simulink model "HarmMultisine_sim"  (R2019b)
settings: Solver=VariableStepAuto  StartTime=0.0  StopTime=10.0  RelTol=1e-3
settings Model: Creator=s164234  LastModifiedBy=s164234

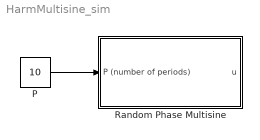
== system HarmMultisine_sim ==
  P : Constant  Value=10
  "Random Phase Multisine " : Subsystem
  wires:
  P/1 -> "Random Phase Multisine "/1("P (number of periods) ")

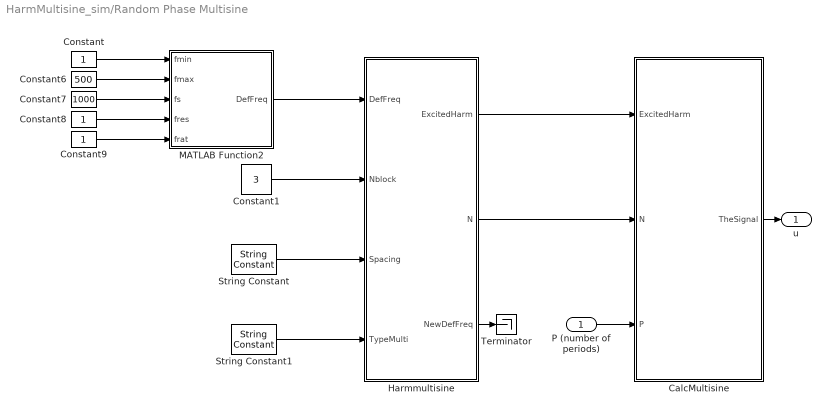
== system HarmMultisine_sim/Random Phase Multisine  ==
  "P (number of periods) " : Inport
  "CalcMultisine " : MATLAB Function  TreatAsAtomicUnit=on
  Constant : Constant
  Constant1 : Constant  Value=3
  Constant6 : Constant  Value=500
  Constant7 : Constant  Value=1000
  Constant8 : Constant
  Constant9 : Constant
  "Harmmultisine " : MATLAB Function  TreatAsAtomicUnit=on
  MATLAB Function2 : MATLAB Function  TreatAsAtomicUnit=on
  String Constant : StringConstant  String='log'
  String Constant1 : StringConstant  String='full'
  Terminator : Terminator
  u : Outport
  wires:
  "Harmmultisine "/2(N) -> "CalcMultisine "/2(N)
  Constant9/1 -> MATLAB Function2/5(frat)
  String Constant1/1 -> "Harmmultisine "/4(TypeMulti)
  Constant1/1 -> "Harmmultisine "/2(Nblock)
  Constant/1 -> MATLAB Function2/1(fmin)
  Constant7/1 -> MATLAB Function2/3(fs)
  String Constant/1 -> "Harmmultisine "/3(Spacing)
  "CalcMultisine "/1(TheSignal) -> u/1
  Constant6/1 -> MATLAB Function2/2(fmax)
  "Harmmultisine "/1(ExcitedHarm) -> "CalcMultisine "/1(ExcitedHarm)
  Constant8/1 -> MATLAB Function2/4(fres)
  MATLAB Function2/1(DefFreq) -> "Harmmultisine "/1(DefFreq)
  "P (number of periods) "/1 -> "CalcMultisine "/3(P)
  "Harmmultisine "/3(NewDefFreq) -> Terminator/1

== matlab function HarmMultisine_sim/Random Phase Multisine /Harmmultisine  ==
  data: DefFreq input; ExcitedHarm output; Nblock input; Spacing input; TypeMulti input; N output; NewDefFreq output
function [ExcitedHarm, N, NewDefFreq] = HarmMultisine(DefFreq, Nblock, Spacing, TypeMulti)
%
%       function [ExcitedHarm, N, NewDefFreq] = HarmMultisine(DefFreq, Nblock, Spacing, TypeMulti);
%
%       calculates the harmonic content of an odd or full random harmonic grid multisine signal
%       with a linear or a logarithmic spacing in the band defined by [fmin, fmax]
%       for a lowpass design
%           fmin = fres/2	for odd multisines
%           fmin = fres     for full multisines
%       where
%           fres =          the frequency spacing between two consecutive odd harmonics for odd multisines 
%           fres =          the frequency spacing between two consecutive harmonics for full multisines 
%
%
%   OUTPUT
%
%       ExcitedHarm     =   excited frequencies of the multisine expressed in harmonic numbers
%
%       N               =   number of time domain samples in one period
%
%       NewDefFreq      =   struct containing the information about the sampling frequency, frequency resolution,
%                           and the excited frequency band {'fs', 'fmin', 'fmax', 'fres', 'frat'}
%                               NewDefFreq.fs      =    sampling frequency of the generator (remains unchanged!)
%                               NewDefFreq.fres    =    frequency spacing in Hz between the (odd) harmonics 
%                                                       fres is modified such that fs/fres is an integer number
%                                                       Note: not all (odd) harmonics are excited; especially for the log spacing
%                               NewDefFreq.fmin    =    lowest excited frequency in Hz
%                                                       fmin is modified such that fmin/fres is an (odd) integer number
%                                                       (for lowpass design fmin = fres/2)
%                               NewDefFreq.fmax    =    largest excited frequency in Hz
%                                                       fmax is modified such that fmax/fres is an (odd) integer number
%
%   INPUT
%
%       DefFreq         =   struct containing the information about the sampling frequency, frequency resolution,
%                           and the excited frequency band {'fs', 'fmin', 'fmax', 'fres', 'frat'}
%                               DefFreq.fs      =   sampling frequency of the generator
%                               DefFreq.fres    =   frequency spacing in Hz between the (odd) harmonics 
%                               DefFreq.fmin    =   lowest excited frequency in Hz
%                                                   (for lowpass design of odd multisines fmin = fres/2)
%                               DefFreq.fmax    =   largest excited frequency in Hz
%                               DefFreq.frat    =   ratio between consecutive (odd) harmonics for a logarithmic frequency spacing
%
%       Nblock          =   size of the group of consecutive (odd) harmonics where one is randomly eliminated
%                           if Nblock = Inf then no detection lines are present 
%
%       Spacing         =   linear or logarithmic frequency spacing; optional parameter (default = 'linear') 
%                               'lin', 'linear':       linear frequency spacing
%                               'log', 'logarithmic':  quasi logarithmic frequency spacing (rounded to DFT grid)
%
%       TypeMulti       =   type multisine; optional (default = 'odd')
%                               'odd':   odd random harmonic grid multisine        
%                               'full':  full random harmonic grid multisine 
%
% Copyright (c) Rik Pintelon, Vrije Universiteit Brussel - dept. ELEC, March 2006 
% All rights reserved.
% Software can be used freely for non-commercial applications only.
% Version 4 December 2007
%

%%%%%%%%%%%%%%%%%%%%%%%%%%%%
% initialize the variables %
%%%%%%%%%%%%%%%%%%%%%%%%%%%%

fs = DefFreq.fs;
fres = DefFreq.fres;
fmin = DefFreq.fmin;
fmax = DefFreq.fmax;

if isfield(DefFreq, 'frat')
	if ~isempty(DefFreq.frat)
        frat = DefFreq.frat;
	end % if not empty
end % if isfield

% type of the frequency spacing
if nargin == 2
    Spacing = 'lin';
end % if
Spacing = lower(Spacing);

% type of the multisine
if nargin <= 3
    TypeMulti = 'odd';
end % if
TypeMulti = lower(TypeMulti);


%%%%%%%%%%%%%%%%%%%%%%%%%%%%%%%%%%%%%%%%
% calculation odd random harmonic grid %
%%%%%%%%%%%%%%%%%%%%%%%%%%%%%%%%%%%%%%%%

if strcmp(TypeMulti, 'odd')
    fres = fres/2;                  % frequency spacing between odd and even harmonics
end % if odd multisine
N = ceil(fs/fres);                  % number of time domain points in one period
fres = fs/N;
FreqSpan = floor(fmax/fres);        % frequency span for a lowpass signal

% calculate the (odd) random harmonic numbers for a lowpass signal
switch Spacing
    
    case {'lin', 'linear'}				
		ExcitedHarm = lintone(FreqSpan, Nblock, TypeMulti);
		
    case {'log', 'logarithmic'}
        ExcitedHarm = logtone(FreqSpan, frat, Nblock, TypeMulti);
        
end % switch Spacing

% convert lowpass in bandpass
FirstNonZeroHarm = ceil(fmin/fres);
RemoveHarm = find(ExcitedHarm < FirstNonZeroHarm);
ExcitedHarm(RemoveHarm) = [];


%%%%%%%%%%%%%%%%%%%%%%%%
% realised frequencies %
%%%%%%%%%%%%%%%%%%%%%%%%

NewDefFreq.fs = fs;
NewDefFreq.fres = fres;
if strcmp(TypeMulti, 'odd')
    NewDefFreq.fres = 2*NewDefFreq.fres;       % frequency spacing between the odd harmonics
end % if odd multisine
NewDefFreq.fmin = ExcitedHarm(1)*fres;
NewDefFreq.fmax = ExcitedHarm(end)*fres;

function ExcitedHarm = logtone(FreqSpan, FreqRatio, Nblock, TypeMulti);
%
%	ExcitedHarm = logtone(FreqSpan, FreqRatio, Nblock, TypeMulti);
%
%		(odd) multisine with logaritmic frequency distribution and randomly
%		distributed (odd) detection lines.
%		calculates a logarithmic distributed frequency grid of (odd) harmonics
%		where one (odd) harmonic out of Nblock consecutive harmonics is left out		
%
%	OUTPUT PARAMETERS
%
%		ExcitedHarm		= vector containing the excited harmonics
%
%	INPUT PARAMETERS
%
%		FreqSpan		=   ratio fmax/fmin
%		FreqRatio		=   ratio consecutive odd frequencies in logtone
% 		Nblock			=   number of lines per block
%                           if Nblock = Inf then no detection lines are present 
%       TypeMulti       =   type multisine; optional (default = 'odd')
%                               'odd':   odd random harmonic grid multisine        
%                               'full':  full random harmonic grid multisine 
%
% Johan Schoukens and Rik Pintelon, September 2003
% Version March 18, 2008
%

% type of the multisine
if nargin == 3
    TypeMulti = 'odd';
end % if
TypeMulti = lower(TypeMulti);

% selection of the frequency span
switch TypeMulti    
    case 'odd', Fmax = FreqSpan/2;
    case 'full', Fmax = FreqSpan;        
end % switch

% resolution of the frequency axis = fmin 
% => total number of frequencies on the linear grid = FreqSpan = fmax/fmin

freqv = [1:Fmax];
ExcitedHarm = lin2log(freqv, FreqRatio);		% generates a full quasi log frequency grid

if ~isinf(Nblock)
    Nlog = length(ExcitedHarm);
    NEmpty = floor((Nlog-Nblock)/Nblock);			% number of detection lines 
    ss = floor(Nblock*rand(NEmpty+1,1)) + 1;        % random choice of integer numbers from 1:1:Nblock
    dummy = [0:NEmpty]'*Nblock + ss;
    ExcitedHarm(dummy) = [];
end % if not Nblock = inf

if strcmp(TypeMulti, 'odd')
    ExcitedHarm = 2*ExcitedHarm - 1;			% no even harmonics
end % if odd multisine

== matlab function HarmMultisine_sim/Random Phase Multisine /CalcMultisine  ==
  data: ExcitedHarm input; TheSignal output; N input; P input
function TheSignal = CalcMultisine(ExcitedHarm, N, P)
%
%       TheSignal = CalcMultisine(ExcitedHarm, N, AmplExcitedHarm)
%
%       Calculates one period of a random phase multisine with rms value equal to 1
%
%   OUTPUT
%       TheSignal           =	one period of the time domain signal
%                               rms value equals one 
%
%   INPUT
%       ExcitedHarm         =	excited harmonics of the multisine expressed in harmonic number
%       N                   =	number of time domain samples in one period
%       AmplExcitedHarm     =   optional parameter: amplitudes of the excited harmonics; 
%                               default value: uniform
%
% Copyright (c) Rik Pintelon, Vrije Universiteit Brussel - dept. ELEC, March 2006 
% All rights reserved.
% Software can be used freely for non-commercial applications only.
% Version October 2009
%


% calculation time domain signal
S = zeros(N,1);
S(ExcitedHarm + 1) = ones(size(ExcitedHarm)) .* exp(sqrt(-1)*2*pi*rand(size(ExcitedHarm)));
TheSignal = 2*real(ifft(S));
TheSignal = TheSignal/rms(TheSignal);  % rms value = 1

u = u1 = repmat(TheSignal,P,1);

== matlab function HarmMultisine_sim/Random Phase Multisine /MATLAB Function2 ==
  data: fmin input; DefFreq output; fmax input; fs input; fres input; frat input
function DefFreq = fcn(fmin, fmax, fs, fres, frat)

DefFreq.fmin = fmin;
DefFreq.fmax = fmax;
DefFreq.fs = fs;
DefFreq.fres = fres;
DefFreq.frat = frat;
